simulink model "dynamic_center_out"  (Simulink 8.0)
settings: Solver=FixedStepDiscrete  StartTime=0.0  StopTime=Inf  FixedStep=.001  RelTol=1e-3
libraries: limblab x10, xpclib x3, IntelSMIlibR2007b x1
CloseFcn:
  | rtwprivate ssgencode ModelCloseRequest rwalk_multi_local_v1
settings Model: Creator=limblab  LastModifiedBy=system administrator  ParamWorkspaceSource=ReferencedWorkspace  ExtModeArmWhenConnect=off  BufferReuse=off
settings DataIOCC: LimitDataPoints=off  SaveFormat=StructureWithTime  SignalLoggingSaveFormat=ModelDataLogs  SaveState=on  SignalLoggingName=sigsOut
settings OptimizationCC: BlockReduction=off  BooleanDataType=off  OptimizeBlockIOStorage=off  BufferReuse=off  ExpressionFolding=off  FoldNonRolledExpr=off  LocalBlockOutputs=off  InitFltsAndDblsToZero=on
settings DebuggingCC: SaveWithParameterizedLinksMsg=none  SignalResolutionControl=TryResolveAllWithWarning  SolverPrmCheckMsg=none  MultiTaskDSMMsg=warning  MultiTaskCondExecSysMsg=none  FcnCallInpInsideContextMsg=UseLocalSettings  StrictBusMsg=None
settings HardwareCC: ProdIntDivRoundTo=Zero  ProdEndianess=LittleEndian  ProdHWDeviceType=Generic->32-bit x86 compatible  TargetIntDivRoundTo=Floor  TargetEndianess=LittleEndian  TargetHWDeviceType=32-bit xPC Target (Intel Pentium)
settings SFSimCC: SimParseCustomCode=off
settings RTWCC: SystemTargetFile=xpctarget.tlc  TemplateMakefile=xpc_default_tmf  Description=xPC Target  GenerateReport=on  ProcessScript=xpctarget_make_rtw_hook  CustomSource=targets.c  IncludeERTFirstTime=on  RTWCompilerOptimization=On
settings xpcTargetCC: TargetFcnLib=ansi_tfl_tmw.mat  CodeReplacementLibrary=XPC_BLAS  ParMdlRefBuildCompliant=on  ConcurrentExecutionCompliant=on  CombineSignalStateStructs=off  GRTInterface=on  xPCTaskExecutionProfile=off  xPCRL32EventNumber=5000  xPCisDownloadable=off  xPCLoadParamSetFile=off  xPCConcurrentTasks=off  xPCEnableSFAnimation=off

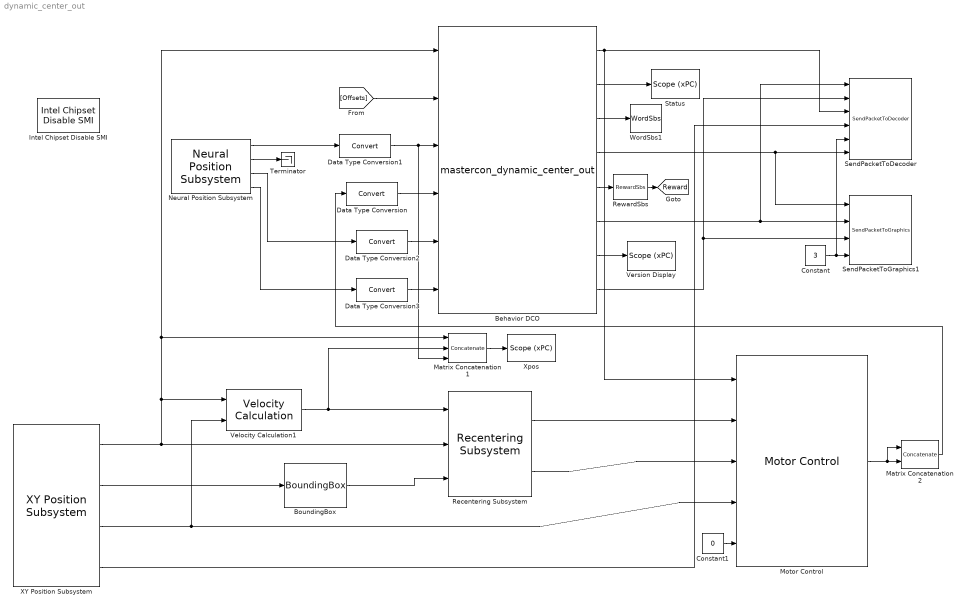
== system dynamic_center_out ==
  Behavior DCO : S-Function  FunctionName=mastercon_dynamic_center_out  Parameters="1  .5 1 .5 1 2 2 10  .5 0  3 8 .5 2 0  3 5 10  3 2 4 .1  .5 .1 1  0 0  0  1"  EnableBusSupport=off
      mask Display:
      | disp('Master Control')
      | port_label('input',1,'pos')
      | port_label('input',2,'pos offsets')
      | port_label('input',3,'force')
      | port_label('input',4,'task off')
      | port_label('input',5,'extra 1')
      | port_label('input',6,'extra 2')
      | port_label('output',1,'force')
      | port_label('output',2,'status')
      | port_label('output',3,'word')
      | port_label('output',4,'targets')
      | port_label('output',5,'reward')
      | port_label('output',6,'tone')
      | port_label('output',7,'version')
      | port_label('output',8,'pos')
  BoundingBox : limblab/BoundingBox
  Constant : Constant  Value=3
  Constant1 : Constant  Value=0
  Data Type Conversion{,1..3} (4 alike) : DataTypeConversion
  Intel Chipset Disable SMI : IntelSMIlibR2007b/Intel Chipset Disable SMI
  Matrix Concatenation1 : Concatenate  NumInputs=3
  Matrix Concatenation2 : Concatenate
  Motor Control : limblab/Motor Control
  Neural Position Subsystem : limblab/Neural Position Subsystem
  Recentering Subsystem : limblab/Recentering Subsystem
  RewardSbs : limblab/RewardSbs
  SendPacketToDecoder : limblab/SendPacketToDecoder
  SendPacketToGraphics1 : limblab/SendPacketToGraphics
  Status : xpclib/Misc./Scope (xPC)   scopeno=3  scopetype=Target  autostart=on  viewmode=Numerical  formatstr='%6.0f state,%6.0f rewards,%6.0f aborts,%6.0f failures,%6.0f incompletes'  grid=on  ylimits=[-10,10]  nosamples=10  noprepostsamples=0  interleave=10  triggermode=FreeRun  triggersignal=1  triggerlevel=0.0  triggerslope=Either  triggerscope=1  triggersample=0  filename=data.dat  mode=Lazy  writesize=512  autorestart=off  dynamicfilemode=off  maxwritefilesize=512*1024^2
  Terminator : Terminator
  Velocity Calculation1 : limblab/Velocity Calculation
  Version Display : xpclib/Misc./Scope (xPC)   scopeno=7  scopetype=Target  autostart=on  viewmode=Numerical  formatstr='%6.0f major,%6.0f minor,%6.0f revision,%6.0f build'  grid=on  ylimits=[-10,10]  nosamples=10  noprepostsamples=0  interleave=10  triggermode=FreeRun  triggersignal=1  triggerlevel=0.0  triggerslope=Either  triggerscope=1  triggersample=0  filename=data.dat  mode=Lazy  writesize=512  autorestart=off  dynamicfilemode=off  maxwritefilesize=512*1024^2
  WordSbs1 : limblab/WordSbs
  XY Position Subsystem : limblab/XY Position Subsystem
  Xpos : xpclib/Misc./Scope (xPC)   scopeno=1  scopetype=Target  autostart=on  viewmode=Numerical  formatstr='%15.2f X,%15.2f Y,%15.2f dX,%15.2f dY,%15.2f X(bc),%15.2f Y(bc)'  grid=on  ylimits=[-10,10]  nosamples=10  noprepostsamples=0  interleave=10  triggermode=FreeRun  triggersignal=1  triggerlevel=0.0  triggerslope=Either  triggerscope=1  triggersample=0  filename=data.dat  mode=Lazy  writesize=512  autorestart=off  dynamicfilemode=off  maxwritefilesize=512*1024^2
  tag scope: Reward=global
  wires:
  Velocity Calculation1/1 -> Recentering Subsystem/1, Matrix Concatenation1/2
  XY Position Subsystem/1 -> Recentering Subsystem/2, Velocity Calculation1/1, Matrix Concatenation1/1, Behavior DCO/1
  Behavior DCO/2 -> Status/1
  Behavior DCO/3 -> WordSbs1/1
  Behavior DCO/1 -> SendPacketToDecoder/3, Motor Control/1
  Behavior DCO/5 -> RewardSbs/1
  BoundingBox/1 -> Recentering Subsystem/3
  XY Position Subsystem/3 -> Motor Control/4, Velocity Calculation1/2
  XY Position Subsystem/2 -> BoundingBox/1
  Matrix Concatenation1/1 -> Xpos/1
  Recentering Subsystem/2 -> Motor Control/3
  Recentering Subsystem/1 -> Motor Control/2
  RewardSbs/1 -> [Reward]
  Constant/1 -> SendPacketToDecoder/5, SendPacketToGraphics1/4
  Behavior DCO/4 -> SendPacketToGraphics1/1, SendPacketToDecoder/6
  [Offsets] -> Behavior DCO/2
  Behavior DCO/6 -> SendPacketToGraphics1/2, SendPacketToDecoder/1
  Behavior DCO/7 -> Version Display/1
  Behavior DCO/8 -> SendPacketToGraphics1/3, SendPacketToDecoder/2
  Motor Control/1 -> Matrix Concatenation2/1, Matrix Concatenation2/2
  Matrix Concatenation2/1 -> Data Type Conversion/1
  Data Type Conversion/1 -> Behavior DCO/4
  Constant1/1 -> Motor Control/5
  Neural Position Subsystem/1 -> Data Type Conversion1/1
  Neural Position Subsystem/2 -> Terminator/1
  Data Type Conversion1/1 -> Matrix Concatenation1/3, Behavior DCO/3
  Neural Position Subsystem/4 -> Data Type Conversion3/1
  Data Type Conversion3/1 -> Behavior DCO/6
  Data Type Conversion2/1 -> Behavior DCO/5
  Neural Position Subsystem/3 -> Data Type Conversion2/1
  XY Position Subsystem/4 -> SendPacketToDecoder/4
